simulink model "vectorBus"  (R2024a)
settings: Solver=VariableStepAuto  StartTime=0.0  StopTime=10.0  RelTol=1e-3
settings Model: Creator=bneiswan  LastModifiedBy=bneiswan
settings RTWCC: GPUComputeCapability=3.5

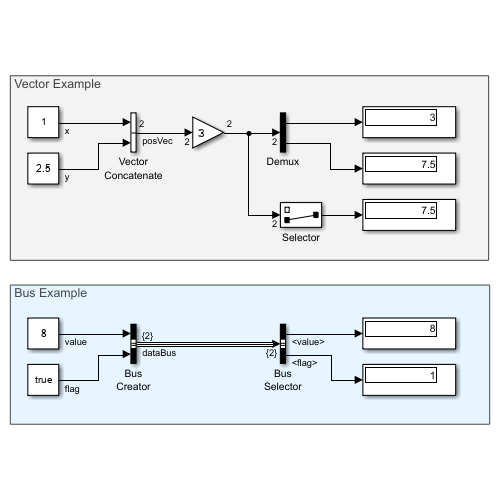
[thumbnail: Simulink's stored preview of the top-level diagram]
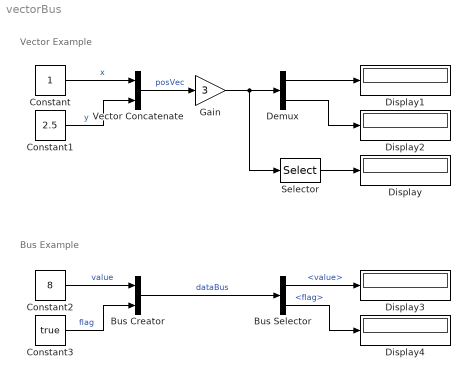
== system vectorBus ==
  note: Bus Example
  note: Vector Example
  Bus Creator : BusCreator  Inputs=2
  Bus Selector : BusSelector  OutputSignals=value,flag
  Constant : Constant  OutDataTypeStr=double
  Constant1 : Constant  Value=2.5  OutDataTypeStr=double
  Constant2 : Constant  Value=8  OutDataTypeStr=double
  Constant3 : Constant  Value=true  OutDataTypeStr=boolean
  Demux : Demux  Outputs=2
  Display{,1..4} (5 alike) : Display
  Gain : Gain  Gain=3
  Selector : Selector  InputPortWidth=2  IndexOptions=Index vector (dialog)  Indices=2  OutputSizes=1
  Vector Concatenate : Concatenate
  wires:
  Vector Concatenate/1 -> Gain/1  "posVec"
  Demux/2 -> Display2/1
  Bus Selector/2 -> Display4/1  "<flag>"
  Bus Selector/1 -> Display3/1  "<value>"
  Demux/1 -> Display1/1
  Constant3/1 -> Bus Creator/2  "flag"
  Selector/1 -> Display/1
  Gain/1 -> Demux/1, Selector/1
  Constant/1 -> Vector Concatenate/1  "x"
  Bus Creator/1 -> Bus Selector/1  "dataBus"
  Constant1/1 -> Vector Concatenate/2  "y"
  Constant2/1 -> Bus Creator/1  "value"
